simulink model "pkt1"  (R2013a)
settings: Solver=ode45  SolverMode=SingleTasking  StartTime=0.0  StopTime=8  RelTol=1e-3
undefined symbols (not defined in the file): B, psi_e, Rt, T
settings Model: Creator=konra  LastModifiedBy=Wojciech
settings DataIOCC: SignalLoggingSaveFormat=ModelDataLogs
settings OptimizationCC: BlockReduction=off  BooleanDataType=off
settings DebuggingCC: SaveWithParameterizedLinksMsg=none  SignalResolutionControl=TryResolveAllWithWarning  SolverPrmCheckMsg=none  MultiTaskDSMMsg=warning  MultiTaskCondExecSysMsg=none  StrictBusMsg=None
settings HardwareCC: TargetUnknown=on
settings RTWCC: IncludeERTFirstTime=on

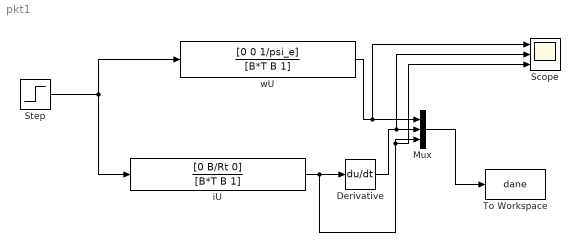
== system pkt1 ==
  Derivative : Derivative
  Mux : Mux  Inputs=3
  Scope : Scope  NumInputPorts=3
      settings: YMin=-5~-5~-5  YMax=5~5~5
  Step : Step  After=220  SampleTime=0
  To Workspace : ToWorkspace  VariableName=dane  SampleTime=-1  SaveFormat=Structure With Time
  iU : TransferFcn  Numerator=[0 B/Rt 0]  Denominator=[B*T B 1]
  wU : TransferFcn  Numerator=[0 0 1/psi_e]  Denominator=[B*T B 1]
  wires:
  wU/1 -> Scope/1, Mux/1
  Step/1 -> wU/1, iU/1
  Derivative/1 -> Scope/2, Mux/2
  Mux/1 -> To Workspace/1
  iU/1 -> Scope/3, Mux/3, Derivative/1
